simulink model "Block"  (R2014b)
settings: Solver=ode45  StartTime=0.0  StopTime=10.0  RelTol=1e-3
settings Model: Creator=99641  LastModifiedBy=99641

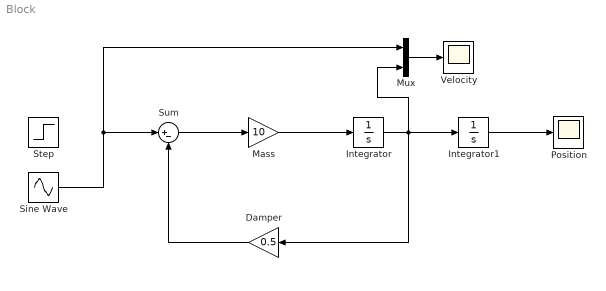
== system Block ==
  Damper : Gain  Gain=0.5
  Integrator : Integrator
  Integrator1 : Integrator
  Mass : Gain  Gain=10
  Mux : Mux  Inputs=2
  "Position " : Scope
  Sine Wave : Sin  SampleTime=0
  Step : Step  SampleTime=0
  Sum : Sum  Inputs=|+-
  Velocity : Scope
  wires:
  Sum/1 -> Mass/1
  Integrator1/1 -> "Position "/1
  Damper/1 -> Sum/2
  Sine Wave/1 -> Mux/1, Sum/1
  Mux/1 -> Velocity/1
  Integrator/1 -> Mux/2, Damper/1, Integrator1/1
  Mass/1 -> Integrator/1
